simulink model "SistemaLinealFuzzy"  (R2018b)
settings: Solver=VariableStepAuto  StartTime=0.0  StopTime=ttotal  RelTol=1e-3
values from neighbouring files (symbols this model uses):
  iseed = randi(2^53-1)    [IdentificacionTS.m]
  tmuestra = 0.2    [ControlDeEstadosTS.m]    (also in IdentificacionTS.m = 0.02; MultiTestTS.m = 0.02)
undefined symbols (not defined in the file or in its folder): Borrosolinealmagia, denom1, denom2, denom3, num1, num2, num3
settings Model: Creator=pablo  LastModifiedBy=pablo

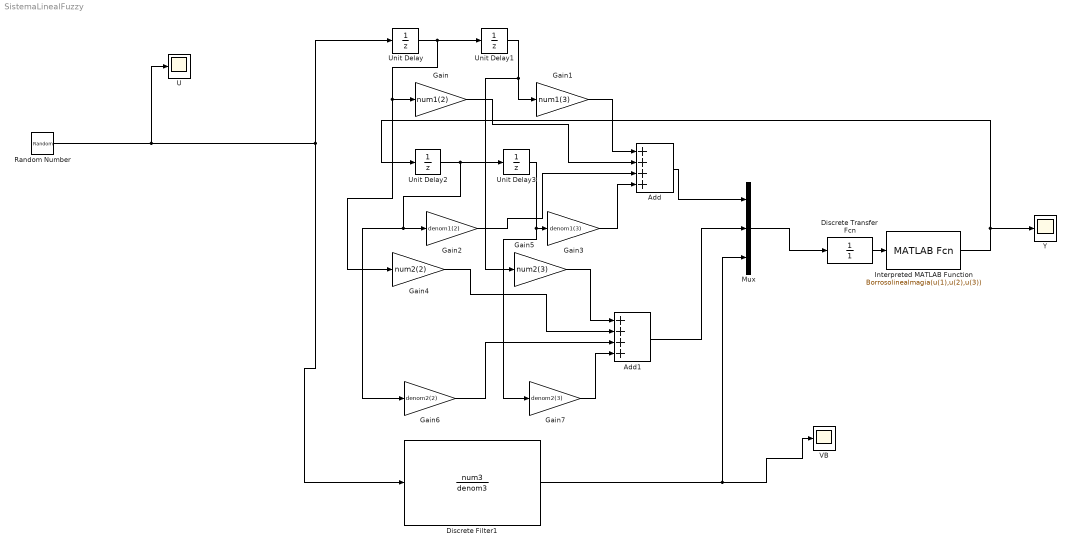
== system SistemaLinealFuzzy ==
  Add : Sum  Inputs=4
  Add1 : Sum  Inputs=4
  Discrete Transfer Fcn : DiscreteTransferFcn  Denominator=[1]  SampleTime=tmuestra
  Discrete Filter1 : DiscreteFilter  Numerator=num3  Denominator=denom3  SampleTime=tmuestra
  Gain : Gain  Gain=num1(2)
  Gain1 : Gain  Gain=num1(3)
  Gain2 : Gain  Gain=denom1(2)
  Gain3 : Gain  Gain=denom1(3)
  Gain4 : Gain  Gain=num2(2)
  Gain5 : Gain  Gain=num2(3)
  Gain6 : Gain  Gain=denom2(2)
  Gain7 : Gain  Gain=denom2(3)
  Interpreted MATLAB Function : MATLABFcn  MATLABFcn=Borrosolinealmagia(u(1),u(2),u(3))  OutputDimensions=1
  Mux : Mux  Inputs=3
  Random Number : RandomNumber  Variance=0.05  Seed=iseed  SampleTime=tmuestra
  "U " : Scope
  Unit Delay{,1..3} (4 alike) : UnitDelay  SampleTime=-1
  VB : Scope
  "Y " : Scope
  wires:
  Random Number/1 -> Unit Delay/1, Discrete Filter1/1, "U "/1
  Add1/1 -> Mux/2
  Discrete Filter1/1 -> VB/1, Mux/3
  Interpreted MATLAB Function/1 -> "Y "/1, Unit Delay2/1
  Mux/1 -> Discrete Transfer Fcn/1
  Discrete Transfer Fcn/1 -> Interpreted MATLAB Function/1
  Unit Delay/1 -> Gain4/1, Gain/1, Unit Delay1/1
  Unit Delay1/1 -> Gain1/1, Gain5/1
  Unit Delay3/1 -> Gain7/1, Gain3/1
  Gain/1 -> Add/2
  Gain1/1 -> Add/1
  Gain2/1 -> Add/3
  Gain3/1 -> Add/4
  Add/1 -> Mux/1
  Gain7/1 -> Add1/4
  Gain4/1 -> Add1/2
  Gain6/1 -> Add1/3
  Gain5/1 -> Add1/1
  Unit Delay2/1 -> Gain6/1, Gain2/1, Unit Delay3/1
